simulink model "genData"  (R2025b)
settings: Solver=VariableStepAuto  StartTime=0.0  StopTime=10.0  RelTol=1e-3
undefined symbols (not defined in the file or in its folder): init_states_BLACK, init_states_BLUE, init_states_RED
settings Model: Creator=ryan  LastModifiedBy=ryan

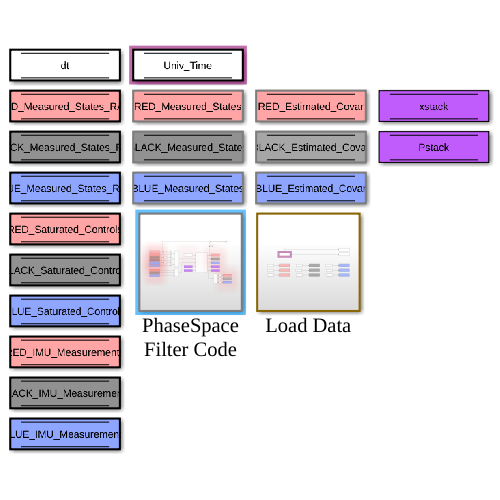
[thumbnail: Simulink's stored preview of the top-level diagram]
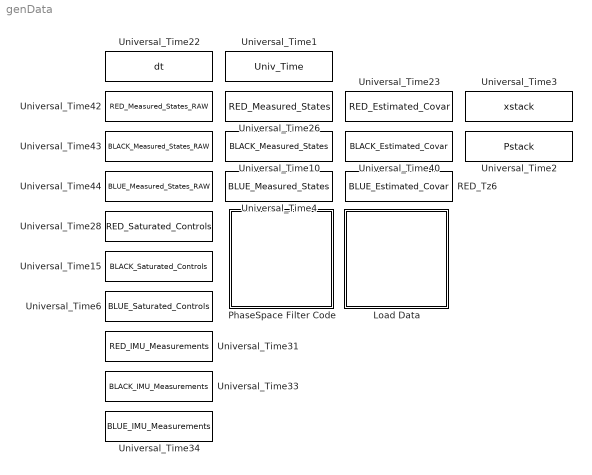
== system genData ==
  Load Data : Subsystem
  PhaseSpace Filter Code : Subsystem
  RED_Tz6 : DataStoreMemory  DataStoreName=BLUE_Estimated_Covar  ReadBeforeWriteMsg=warning  WriteAfterWriteMsg=warning  WriteAfterReadMsg=warning  InitialValue=zeros(6*6,1)  ShowAdditionalParam=off
  Universal_Time1 : DataStoreMemory  DataStoreName=Univ_Time  ReadBeforeWriteMsg=warning  WriteAfterWriteMsg=warning  WriteAfterReadMsg=warning  ShowAdditionalParam=off
  Universal_Time10 : DataStoreMemory  DataStoreName=BLACK_Measured_States  ReadBeforeWriteMsg=warning  WriteAfterWriteMsg=warning  WriteAfterReadMsg=warning  InitialValue=[0;0;0;0;0;0;0;0;0]  ShowAdditionalParam=off
  Universal_Time15 : DataStoreMemory  DataStoreName=BLACK_Saturated_Controls  ReadBeforeWriteMsg=warning  WriteAfterWriteMsg=warning  WriteAfterReadMsg=warning  InitialValue=[0;0;0]  ShowAdditionalParam=off
  Universal_Time2 : DataStoreMemory  DataStoreName=Pstack  ReadBeforeWriteMsg=warning  WriteAfterWriteMsg=warning  WriteAfterReadMsg=warning  InitialValue=zeros(6*6,1)  ShowAdditionalParam=off
  Universal_Time22 : DataStoreMemory  DataStoreName=dt  ReadBeforeWriteMsg=warning  WriteAfterWriteMsg=warning  WriteAfterReadMsg=warning  ShowAdditionalParam=off
  Universal_Time23 : DataStoreMemory  DataStoreName=RED_Estimated_Covar  ReadBeforeWriteMsg=warning  WriteAfterWriteMsg=warning  WriteAfterReadMsg=warning  InitialValue=zeros(6*6,1)  ShowAdditionalParam=off
  Universal_Time26 : DataStoreMemory  DataStoreName=RED_Measured_States  ReadBeforeWriteMsg=warning  WriteAfterWriteMsg=warning  WriteAfterReadMsg=warning  InitialValue=[0;0;0;0;0;0;0;0;0]  ShowAdditionalParam=off
  Universal_Time28 : DataStoreMemory  DataStoreName=RED_Saturated_Controls  ReadBeforeWriteMsg=warning  WriteAfterWriteMsg=warning  WriteAfterReadMsg=warning  InitialValue=[0;0;0]  ShowAdditionalParam=off
  Universal_Time3 : DataStoreMemory  DataStoreName=xstack  ReadBeforeWriteMsg=warning  WriteAfterWriteMsg=warning  WriteAfterReadMsg=warning  InitialValue=zeros(6*6,1)  ShowAdditionalParam=off
  Universal_Time31 : DataStoreMemory  DataStoreName=RED_IMU_Measurements  ReadBeforeWriteMsg=warning  WriteAfterWriteMsg=warning  WriteAfterReadMsg=warning  InitialValue=[0;0;0]  ShowAdditionalParam=off
  Universal_Time33 : DataStoreMemory  DataStoreName=BLACK_IMU_Measurements  ReadBeforeWriteMsg=warning  WriteAfterWriteMsg=warning  WriteAfterReadMsg=warning  InitialValue=[0;0;0]  ShowAdditionalParam=off
  Universal_Time34 : DataStoreMemory  DataStoreName=BLUE_IMU_Measurements  ReadBeforeWriteMsg=warning  WriteAfterWriteMsg=warning  WriteAfterReadMsg=warning  InitialValue=[0;0;0]  ShowAdditionalParam=off
  Universal_Time4 : DataStoreMemory  DataStoreName=BLUE_Measured_States  ReadBeforeWriteMsg=warning  WriteAfterWriteMsg=warning  WriteAfterReadMsg=warning  InitialValue=[0;0;0;0;0;0;0;0;0]  ShowAdditionalParam=off
  Universal_Time40 : DataStoreMemory  DataStoreName=BLACK_Estimated_Covar  ReadBeforeWriteMsg=warning  WriteAfterWriteMsg=warning  WriteAfterReadMsg=warning  InitialValue=zeros(6*6,1)  ShowAdditionalParam=off
  Universal_Time42 : DataStoreMemory  DataStoreName=RED_Measured_States_RAW  ReadBeforeWriteMsg=warning  WriteAfterWriteMsg=warning  WriteAfterReadMsg=warning  InitialValue=[init_states_RED';0;0;0;0;0;0]  ShowAdditionalParam=off
  Universal_Time43 : DataStoreMemory  DataStoreName=BLACK_Measured_States_RAW  ReadBeforeWriteMsg=warning  WriteAfterWriteMsg=warning  WriteAfterReadMsg=warning  InitialValue=[init_states_BLACK';0;0;0;0;0;0]  ShowAdditionalParam=off
  Universal_Time44 : DataStoreMemory  DataStoreName=BLUE_Measured_States_RAW  ReadBeforeWriteMsg=warning  WriteAfterWriteMsg=warning  WriteAfterReadMsg=warning  InitialValue=[init_states_BLUE';0;0;0;0;0;0]  ShowAdditionalParam=off
  Universal_Time6 : DataStoreMemory  DataStoreName=BLUE_Saturated_Controls  ReadBeforeWriteMsg=warning  WriteAfterWriteMsg=warning  WriteAfterReadMsg=warning  InitialValue=[0;0;0]  ShowAdditionalParam=off

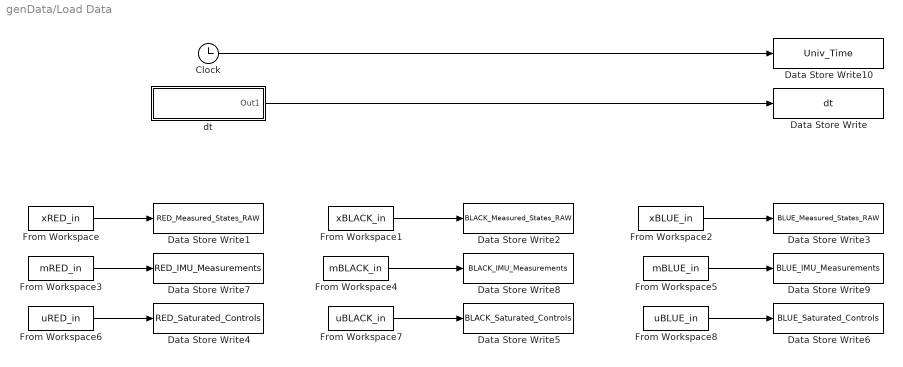
== system genData/Load Data ==
  Clock : Clock
  Data Store Write : DataStoreWrite  DataStoreName=dt  IndexOptions=Index vector (dialog)  Indices=1  OutputSizes=1
  Data Store Write1 : DataStoreWrite  DataStoreName=RED_Measured_States_RAW  IndexOptions=Index vector (dialog)  Indices=1  OutputSizes=1
  Data Store Write10 : DataStoreWrite  DataStoreName=Univ_Time  IndexOptions=Index vector (dialog)  Indices=1  OutputSizes=1
  Data Store Write2 : DataStoreWrite  DataStoreName=BLACK_Measured_States_RAW  IndexOptions=Index vector (dialog)  Indices=1  OutputSizes=1
  Data Store Write3 : DataStoreWrite  DataStoreName=BLUE_Measured_States_RAW  IndexOptions=Index vector (dialog)  Indices=1  OutputSizes=1
  Data Store Write4 : DataStoreWrite  DataStoreName=RED_Saturated_Controls  IndexOptions=Index vector (dialog)  Indices=1  OutputSizes=1
  Data Store Write5 : DataStoreWrite  DataStoreName=BLACK_Saturated_Controls  IndexOptions=Index vector (dialog)  Indices=1  OutputSizes=1
  Data Store Write6 : DataStoreWrite  DataStoreName=BLUE_Saturated_Controls  IndexOptions=Index vector (dialog)  Indices=1  OutputSizes=1
  Data Store Write7 : DataStoreWrite  DataStoreName=RED_IMU_Measurements  IndexOptions=Index vector (dialog)  Indices=1  OutputSizes=1
  Data Store Write8 : DataStoreWrite  DataStoreName=BLACK_IMU_Measurements  IndexOptions=Index vector (dialog)  Indices=1  OutputSizes=1
  Data Store Write9 : DataStoreWrite  DataStoreName=BLUE_IMU_Measurements  IndexOptions=Index vector (dialog)  Indices=1  OutputSizes=1
  From Workspace : FromWorkspace  VariableName=xRED_in
  From Workspace1 : FromWorkspace  VariableName=xBLACK_in
  From Workspace2 : FromWorkspace  VariableName=xBLUE_in
  From Workspace3 : FromWorkspace  VariableName=mRED_in
  From Workspace4 : FromWorkspace  VariableName=mBLACK_in
  From Workspace5 : FromWorkspace  VariableName=mBLUE_in
  From Workspace6 : FromWorkspace  VariableName=uRED_in
  From Workspace7 : FromWorkspace  VariableName=uBLACK_in
  From Workspace8 : FromWorkspace  VariableName=uBLUE_in
  dt : Subsystem
  wires:
  dt/1(Out1) -> Data Store Write/1
  From Workspace/1 -> Data Store Write1/1
  From Workspace1/1 -> Data Store Write2/1
  From Workspace2/1 -> Data Store Write3/1
  From Workspace3/1 -> Data Store Write7/1
  From Workspace4/1 -> Data Store Write8/1
  From Workspace5/1 -> Data Store Write9/1
  From Workspace6/1 -> Data Store Write4/1
  From Workspace7/1 -> Data Store Write5/1
  From Workspace8/1 -> Data Store Write6/1
  Clock/1 -> Data Store Write10/1

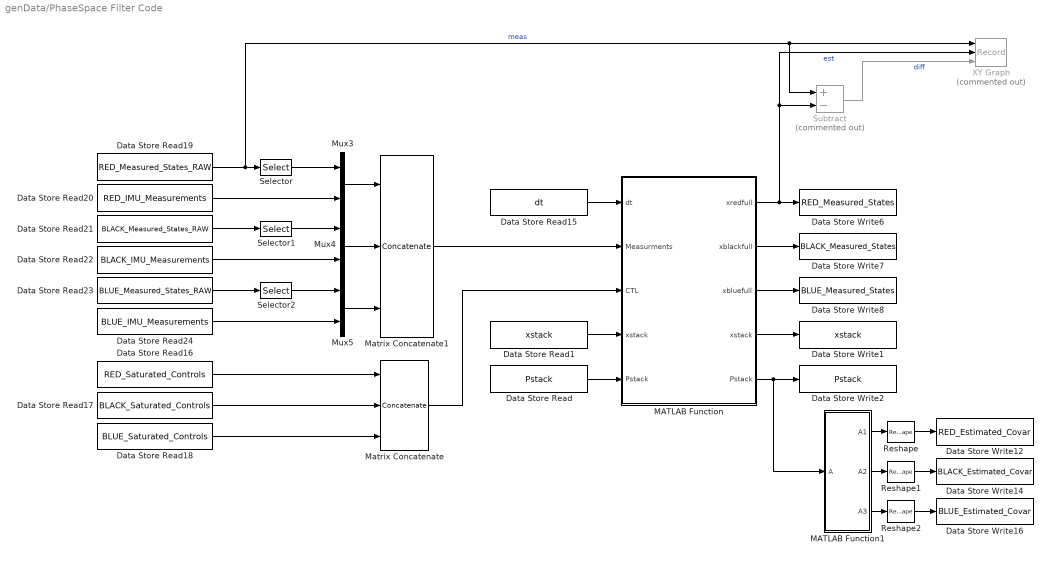
== system genData/PhaseSpace Filter Code ==
  Data Store Read : DataStoreRead  DataStoreName=Pstack  IndexOptions=Index vector (dialog)  Indices=1  OutputSizes=1
  Data Store Read1 : DataStoreRead  DataStoreName=xstack  IndexOptions=Index vector (dialog)  Indices=1  OutputSizes=1
  Data Store Read15 : DataStoreRead  DataStoreName=dt  IndexOptions=Index vector (dialog)  Indices=1  OutputSizes=1
  Data Store Read16 : DataStoreRead  DataStoreName=RED_Saturated_Controls  IndexOptions=Index vector (dialog)  Indices=1  OutputSizes=1
  Data Store Read17 : DataStoreRead  DataStoreName=BLACK_Saturated_Controls  IndexOptions=Index vector (dialog)  Indices=1  OutputSizes=1
  Data Store Read18 : DataStoreRead  DataStoreName=BLUE_Saturated_Controls  IndexOptions=Index vector (dialog)  Indices=1  OutputSizes=1
  Data Store Read19 : DataStoreRead  DataStoreName=RED_Measured_States_RAW  IndexOptions=Index vector (dialog)  Indices=1  OutputSizes=1
  Data Store Read20 : DataStoreRead  DataStoreName=RED_IMU_Measurements  IndexOptions=Index vector (dialog)  Indices=1  OutputSizes=1
  Data Store Read21 : DataStoreRead  DataStoreName=BLACK_Measured_States_RAW  IndexOptions=Index vector (dialog)  Indices=1  OutputSizes=1
  Data Store Read22 : DataStoreRead  DataStoreName=BLACK_IMU_Measurements  IndexOptions=Index vector (dialog)  Indices=1  OutputSizes=1
  Data Store Read23 : DataStoreRead  DataStoreName=BLUE_Measured_States_RAW  IndexOptions=Index vector (dialog)  Indices=1  OutputSizes=1
  Data Store Read24 : DataStoreRead  DataStoreName=BLUE_IMU_Measurements  IndexOptions=Index vector (dialog)  Indices=1  OutputSizes=1
  Data Store Write1 : DataStoreWrite  DataStoreName=xstack  IndexOptions=Index vector (dialog)  Indices=1  OutputSizes=1
  Data Store Write12 : DataStoreWrite  DataStoreName=RED_Estimated_Covar  IndexOptions=Index vector (dialog)  Indices=1  OutputSizes=1
  Data Store Write14 : DataStoreWrite  DataStoreName=BLACK_Estimated_Covar  IndexOptions=Index vector (dialog)  Indices=1  OutputSizes=1
  Data Store Write16 : DataStoreWrite  DataStoreName=BLUE_Estimated_Covar  IndexOptions=Index vector (dialog)  Indices=1  OutputSizes=1
  Data Store Write2 : DataStoreWrite  DataStoreName=Pstack  IndexOptions=Index vector (dialog)  Indices=1  OutputSizes=1
  Data Store Write6 : DataStoreWrite  DataStoreName=RED_Measured_States  IndexOptions=Index vector (dialog)  Indices=1  OutputSizes=1
  Data Store Write7 : DataStoreWrite  DataStoreName=BLACK_Measured_States  IndexOptions=Index vector (dialog)  Indices=1  OutputSizes=1
  Data Store Write8 : DataStoreWrite  DataStoreName=BLUE_Measured_States  IndexOptions=Index vector (dialog)  Indices=1  OutputSizes=1
  MATLAB Function : MATLAB Function  TreatAsAtomicUnit=on
  MATLAB Function1 : MATLAB Function  TreatAsAtomicUnit=on
  Matrix Concatenate : Concatenate  NumInputs=3  Mode=Multidimensional array  ConcatenateDimension=2
  Matrix Concatenate1 : Concatenate  NumInputs=3  Mode=Multidimensional array  ConcatenateDimension=2
  Mux3 : Mux  Inputs=2
  Mux4 : Mux  Inputs=2
  Mux5 : Mux  Inputs=2
  Reshape : Reshape
  Reshape1 : Reshape
  Reshape2 : Reshape
  Selector : Selector  InputPortWidth=9  IndexOptions=Index vector (dialog)  Indices=[1:3]  OutputSizes=1
  Selector1 : Selector  InputPortWidth=9  IndexOptions=Index vector (dialog)  Indices=[1:3]  OutputSizes=1
  Selector2 : Selector  InputPortWidth=9  IndexOptions=Index vector (dialog)  Indices=[1:3]  OutputSizes=1
  Subtract : Sum  Commented=on  Inputs=+-
  XY Graph : Record  Commented=on  NumPorts=3.0  FileSettingsInternal="{\"entries\":[{\"content\":{\"excelSettings\":{\"content\":{},\"type\":\"Streamout.ExcelSettings\"},\"parquetSettings\":{\"content\":{},\"type\":\"Streamout.ParquetSettings\"}},\"type\":\"Streamout.FileSettingStorage\",\"uuid\":\"\"}],\"packageUris\":[\"http:\\/\\/schema.mathworks.com\\/mf0\\/streamout_blocks\\/R2020a\"],\"version\":\"1.0\"}"  FrameSettings=[0, 0, 0]  Layout=[1 1]  SignalsInternal="{\"entries\":[{\"content\":{},\"type\":\"RecordBlkView.InputSignals\",\"uuid\":\"\"}],\"packageUris\":[\"http:\\/\\/schema.mathworks.com\\/mf0\\/streamout_blocks\\/R2020a\"],\"version\":\"1.0\"}"  VisualizationBindings="{\"sparklinesplugin\":{\"info\":[{\"bindingParametersList\":[],\"subplotID\":1}]}}"  CompatibilityTag=XY
  wires:
  Data Store Read15/1 -> MATLAB Function/1(dt)
  Data Store Read16/1 -> Matrix Concatenate/1
  Data Store Read17/1 -> Matrix Concatenate/2
  Data Store Read18/1 -> Matrix Concatenate/3
  Data Store Read21/1 -> Selector1/1
  Data Store Read22/1 -> Mux4/2
  Data Store Read19/1 -> Subtract/1, XY Graph/1, Selector/1  "meas"
  Data Store Read20/1 -> Mux3/2
  Data Store Read23/1 -> Selector2/1
  Data Store Read24/1 -> Mux5/2
  Mux5/1 -> Matrix Concatenate1/3
  Mux4/1 -> Matrix Concatenate1/2
  Mux3/1 -> Matrix Concatenate1/1
  Matrix Concatenate1/1 -> MATLAB Function/2(Measurments)
  Matrix Concatenate/1 -> MATLAB Function/3(CTL)
  Selector/1 -> Mux3/1
  Selector1/1 -> Mux4/1
  Selector2/1 -> Mux5/1
  MATLAB Function/5(Pstack) -> MATLAB Function1/1(A), Data Store Write2/1
  MATLAB Function/1(xredfull) -> Subtract/2, XY Graph/2, Data Store Write6/1  "est"
  MATLAB Function/2(xblackfull) -> Data Store Write7/1
  MATLAB Function/3(xbluefull) -> Data Store Write8/1
  MATLAB Function1/2(A2) -> Reshape1/1
  MATLAB Function1/3(A3) -> Reshape2/1
  MATLAB Function1/1(A1) -> Reshape/1
  Reshape/1 -> Data Store Write12/1
  Reshape1/1 -> Data Store Write14/1
  Reshape2/1 -> Data Store Write16/1
  Subtract/1 -> XY Graph/3  "diff"
  MATLAB Function/4(xstack) -> Data Store Write1/1
  Data Store Read1/1 -> MATLAB Function/4("xstack ")
  Data Store Read/1 -> MATLAB Function/5("Pstack ")

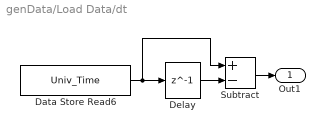
== system genData/Load Data/dt ==
  Data Store Read6 : DataStoreRead  DataStoreName=Univ_Time  IndexOptions=Index vector (dialog)  Indices=1  OutputSizes=1
  Delay : Delay  DelayLength=1  InputProcessing=Columns as channels (frame based)
  Subtract : Sum  Inputs=+-
  Out1 : Outport
  wires:
  Delay/1 -> Subtract/2
  Subtract/1 -> Out1/1
  Data Store Read6/1 -> Subtract/1, Delay/1

== matlab function genData/PhaseSpace Filter Code/MATLAB Function ==
  data: xredfull output; xblackfull output; xbluefull output; xstack output; dt input; Measurments input; CTL input; xstack input; Pstack input; Pstack output; navOpts parameter
function [xredfull, xblackfull, xbluefull, xstack, Pstack] = Navigation(dt, Measurments, CTL, xstack, Pstack, navOpts)
    [xredfull, xblackfull, xbluefull, xstack, Pstack] = spotKF.spotNavigation(dt, Measurments, CTL, xstack, Pstack, navOpts);
end

== matlab function genData/PhaseSpace Filter Code/MATLAB Function1 ==
  data: A input; A1 output; A2 output; A3 output
function [A1,A2,A3] = split3D(A)
%#codegen
A1 = A(:,:,1);
A2 = A(:,:,2);
A3 = A(:,:,3);
end
